simulink subsystem "BrakingHydraulicsDiscBrakesFrontSSC"  (R2025a)
settings: Solver=VariableStepAuto  StartTime=0.0  StopTime=10.0  RelTol=1e-3
undefined symbols (not defined in the file): AxlFL, AxlFR
libraries: sdl_lib x2, nesl_utility_internal x2
settings Model: ModifiedByFormat=The MathWorks, Inc.  Creator=The MathWorks, Inc.  LastModifiedBy=The MathWorks, Inc.
settings OptimizationCC: ReuseModelBlockBuffer=off
settings RTWCC: GPUComputeCapability=3.5  LargeConstantGeneration=WriteOnlyDNNConstantsToDataFiles

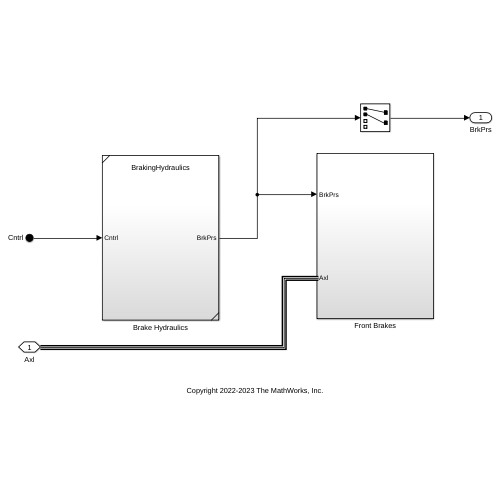
[thumbnail: Simulink's stored preview of the top-level diagram]
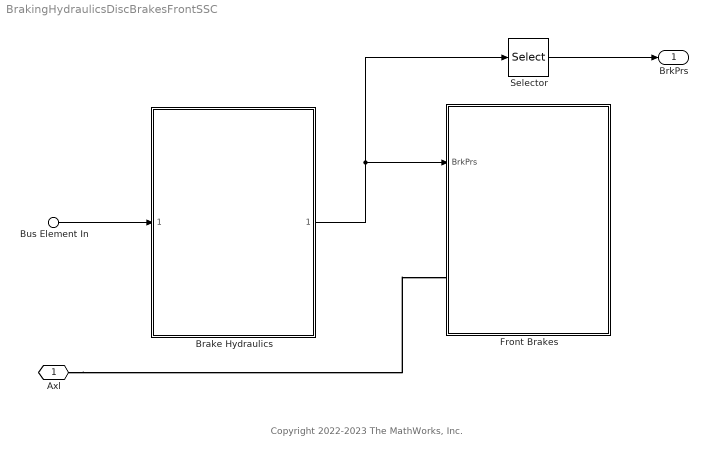
== system BrakingHydraulicsDiscBrakesFrontSSC ==
  note: Copyright 2022-2023 The MathWorks, Inc.
  Bus Element In : Inport  PortName=Cntrl
  Brake Hydraulics : Subsystem  ReferencedSubsystem=BrakingHydraulics
  Front Brakes : Subsystem
  Selector : Selector  InputPortWidth=4  IndexOptions=Index vector (dialog)  Indices=[1 2]  OutputSizes=1
  Axl : PMIOPort  Side=Left
  BrkPrs : Outport  VectorParamsAs1DForOutWhenUnconnected=off
  wires:
  Bus Element In/1 -> Brake Hydraulics/1
  Brake Hydraulics/1 -> Selector/1, Front Brakes/1(BrkPrs)
  Selector/1 -> BrkPrs/1
  connections:
  Axl/RConn1 -- Front Brakes/LConn1

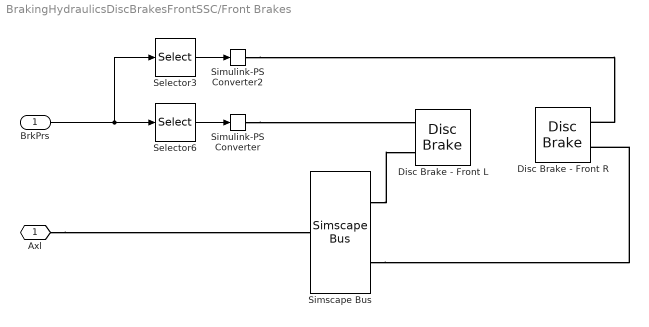
== system BrakingHydraulicsDiscBrakesFrontSSC/Front Brakes ==
  BrkPrs : Inport
  Disc Brake - Front L : sdl_lib/Brakes & Detents/Rotational/Disc Brake  r_mean=PlntBrkPadMeanRadiusFrnt m  bore=PlntBrkActrBoreFrnt m  n_pads=PlntBrkNumPadsFrnt  thermal_port=simscape.enum.thermaleffects.omit  mu_static=PlntBrkStcFricCffFrnt  mu_coulomb=PlntBrkKinFricCffFrnt  temperature_TLU=[280, 300, 320] K  mu_static_TLU=[.9, .8, .7]  mu_coulomb_TLU=[.8, .7, .6]  brkwy_vel=PlntBrkBreakFricVelFrnt rad/s  visc_coef=PlntBrkViscFricFrnt N*m*s/rad  thermal_mass=50 kJ/K  temperature_specify=off  temperature_priority=High  temperature=300 K  temperature_nominal_specify=off  temperature_nominal_value=1  temperature_nominal_unit=K
  Disc Brake - Front R : sdl_lib/Brakes & Detents/Rotational/Disc Brake  r_mean=PlntBrkPadMeanRadiusFrnt m  bore=PlntBrkActrBoreFrnt m  n_pads=PlntBrkNumPadsFrnt  thermal_port=simscape.enum.thermaleffects.omit  mu_static=PlntBrkStcFricCffFrnt  mu_coulomb=PlntBrkKinFricCffFrnt  temperature_TLU=[280, 300, 320] K  mu_static_TLU=[.9, .8, .7]  mu_coulomb_TLU=[.8, .7, .6]  brkwy_vel=PlntBrkBreakFricVelFrnt rad/s  visc_coef=PlntBrkViscFricFrnt N*m*s/rad  thermal_mass=50 kJ/K  temperature_specify=off  temperature_priority=High  temperature=300 K  temperature_nominal_specify=off  temperature_nominal_value=1  temperature_nominal_unit=K
  Selector3 : Selector  InputPortWidth=4  IndexOptions=Index vector (dialog)  Indices=[2]  OutputSizes=1
  Selector6 : Selector  InputPortWidth=4  IndexOptions=Index vector (dialog)  Indices=[1]  OutputSizes=1
  Simscape Bus : SimscapeBus  HierarchyStrings=AxlFL;AxlFR
  Simulink-PS Converter : nesl_utility_internal/Simulink-PS Converter  PhysicalDomain=network_engine_domain  SubClassName=ps_input  LeftPortType=input  RightPortType=output  PseudoPeriodic=off  Frequencies=[]  NoiseDistribution=none  NoiseParameters=[]  Unit=Pa  AffineConversion=off  FilteringAndDerivatives=provide  SimscapeFilterOrder=1  InputFilterTimeConstant=0.001  UdotUserProvided=0
  Simulink-PS Converter2 : nesl_utility_internal/Simulink-PS Converter  PhysicalDomain=network_engine_domain  SubClassName=ps_input  LeftPortType=input  RightPortType=output  PseudoPeriodic=off  Frequencies=[]  NoiseDistribution=none  NoiseParameters=[]  Unit=Pa  AffineConversion=off  FilteringAndDerivatives=provide  SimscapeFilterOrder=1  InputFilterTimeConstant=0.001  UdotUserProvided=0
  Axl : PMIOPort  Side=Left
  wires:
  BrkPrs/1 -> Selector6/1, Selector3/1
  Selector3/1 -> Simulink-PS Converter2/1
  Selector6/1 -> Simulink-PS Converter/1
  connections:
  Simscape Bus/LConn2 -- Disc Brake - Front R/LConn2
  Simulink-PS Converter2/RConn1 -- Disc Brake - Front R/LConn1
  Simulink-PS Converter/RConn1 -- Disc Brake - Front L/LConn1
  Axl/RConn1 -- Simscape Bus/RConn1
  Simscape Bus/LConn1 -- Disc Brake - Front L/LConn2
